simulink model "TuneWall"  (R2025b)
settings: Solver=VariableStepAuto  StartTime=0.0  StopTime=3600*4  RelTol=1e-3
model workspace (MAT data in the model file):
  h_in = 1.419
  h_out = 3.859
  k_Block = 0.01
  k_concrete = 0.11
libraries: fl_lib x66, nesl_utility x19, SimscapeFluids_lib x8
(part 2 of 2)

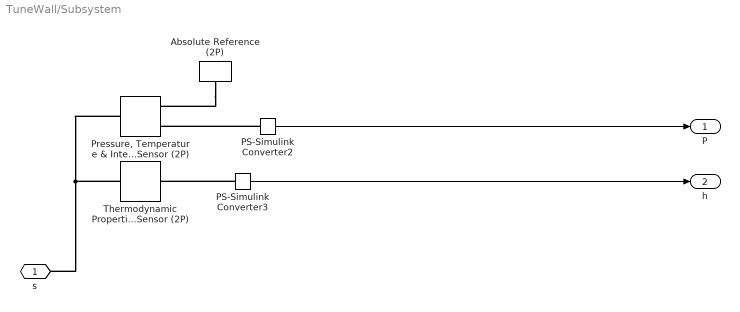
== system TuneWall/Subsystem ==
  Absolute Reference (2P) : fl_lib/Two-Phase Fluid/Elements/Absolute Reference (2P)
  PS-Simulink Converter2 : nesl_utility/PS-Simulink Converter  PhysicalDomain=network_engine_domain  SubClassName=ps_output  LeftPortType=input  RightPortType=output  PseudoPeriodic=off  Frequencies=[]  VectorFormat=inherit  Unit=inherit  AffineConversion=off
  PS-Simulink Converter3 : nesl_utility/PS-Simulink Converter  PhysicalDomain=network_engine_domain  SubClassName=ps_output  LeftPortType=input  RightPortType=output  PseudoPeriodic=off  Frequencies=[]  VectorFormat=inherit  Unit=inherit  AffineConversion=off
  "Pressure, Temperature & Internal Energy Sensor (2P)" : fl_lib/Two-Phase Fluid/Sensors/Pressure, Temperature & Internal Energy Sensor (2P)  reference=foundation.enum.MeasurementReference.difference  pressure=true  pressure_spec=foundation.enum.PressureMeasementSpec.Absolute  temperature=false  internal_energy=false
      settings: InternalSimscapePortConfiguration="{\"Bottom\":[],\"Left\":[{\"id\":\"A\",\"label\":\"A\",\"type\":\"foundation.two_phase_fluid.two_phase_fluid\"}],\"Right\":[{\"id\":\"B\",\"label\":\"B\",\"type\":\"foundation.two_phase_fluid.two_phase_fluid\"},{\"id\":\"P\",\"label\":\"P\",\"type\":\"output\"}],\"Top\":[]}"
  Thermodynamic Properties Sensor (2P) : fl_lib/Two-Phase Fluid/Sensors/Thermodynamic Properties Sensor (2P)  temperature=false  enthalpy=true  density=false  specific_volume=false  entropy=false
      settings: InternalSimscapePortConfiguration="{\"Bottom\":[],\"Left\":[{\"id\":\"A\",\"label\":\"A\",\"type\":\"foundation.two_phase_fluid.two_phase_fluid\"}],\"Right\":[{\"id\":\"H\",\"label\":\"h\",\"type\":\"output\"}],\"Top\":[]}"
  s : PMIOPort  Side=Left
  P : Outport
  h : Outport  Port=2
  wires:
  PS-Simulink Converter3/1 -> h/1
  PS-Simulink Converter2/1 -> P/1
  connections:
  Absolute Reference (2P)/LConn1 -- "Pressure, Temperature & Internal Energy Sensor (2P)"/RConn1
  PS-Simulink Converter2/LConn1 -- "Pressure, Temperature & Internal Energy Sensor (2P)"/RConn2
  PS-Simulink Converter3/LConn1 -- Thermodynamic Properties Sensor (2P)/RConn1
  "Pressure, Temperature & Internal Energy Sensor (2P)"/LConn1 -- s/RConn1 -- Thermodynamic Properties Sensor (2P)/LConn1

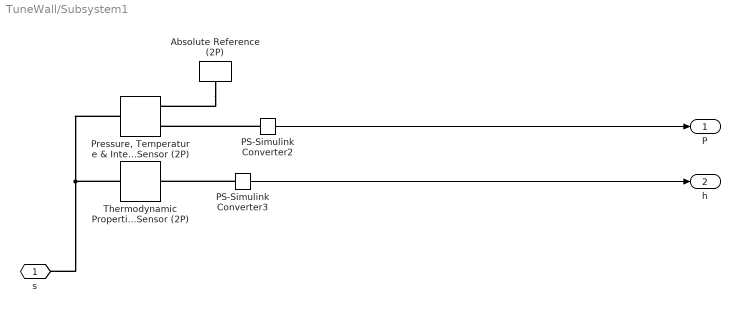
== system TuneWall/Subsystem1 ==
  Absolute Reference (2P) : fl_lib/Two-Phase Fluid/Elements/Absolute Reference (2P)
  PS-Simulink Converter2 : nesl_utility/PS-Simulink Converter  PhysicalDomain=network_engine_domain  SubClassName=ps_output  LeftPortType=input  RightPortType=output  PseudoPeriodic=off  Frequencies=[]  VectorFormat=inherit  Unit=inherit  AffineConversion=off
  PS-Simulink Converter3 : nesl_utility/PS-Simulink Converter  PhysicalDomain=network_engine_domain  SubClassName=ps_output  LeftPortType=input  RightPortType=output  PseudoPeriodic=off  Frequencies=[]  VectorFormat=inherit  Unit=inherit  AffineConversion=off
  "Pressure, Temperature & Internal Energy Sensor (2P)" : fl_lib/Two-Phase Fluid/Sensors/Pressure, Temperature & Internal Energy Sensor (2P)  reference=foundation.enum.MeasurementReference.difference  pressure=true  pressure_spec=foundation.enum.PressureMeasementSpec.Absolute  temperature=false  internal_energy=false
      settings: InternalSimscapePortConfiguration="{\"Bottom\":[],\"Left\":[{\"id\":\"A\",\"label\":\"A\",\"type\":\"foundation.two_phase_fluid.two_phase_fluid\"}],\"Right\":[{\"id\":\"B\",\"label\":\"B\",\"type\":\"foundation.two_phase_fluid.two_phase_fluid\"},{\"id\":\"P\",\"label\":\"P\",\"type\":\"output\"}],\"Top\":[]}"
  Thermodynamic Properties Sensor (2P) : fl_lib/Two-Phase Fluid/Sensors/Thermodynamic Properties Sensor (2P)  temperature=false  enthalpy=true  density=false  specific_volume=false  entropy=false
      settings: InternalSimscapePortConfiguration="{\"Bottom\":[],\"Left\":[{\"id\":\"A\",\"label\":\"A\",\"type\":\"foundation.two_phase_fluid.two_phase_fluid\"}],\"Right\":[{\"id\":\"H\",\"label\":\"h\",\"type\":\"output\"}],\"Top\":[]}"
  s : PMIOPort  Side=Left
  P : Outport
  h : Outport  Port=2
  wires:
  PS-Simulink Converter3/1 -> h/1
  PS-Simulink Converter2/1 -> P/1
  connections:
  Absolute Reference (2P)/LConn1 -- "Pressure, Temperature & Internal Energy Sensor (2P)"/RConn1
  PS-Simulink Converter2/LConn1 -- "Pressure, Temperature & Internal Energy Sensor (2P)"/RConn2
  PS-Simulink Converter3/LConn1 -- Thermodynamic Properties Sensor (2P)/RConn1
  "Pressure, Temperature & Internal Energy Sensor (2P)"/LConn1 -- Thermodynamic Properties Sensor (2P)/LConn1 -- s/RConn1

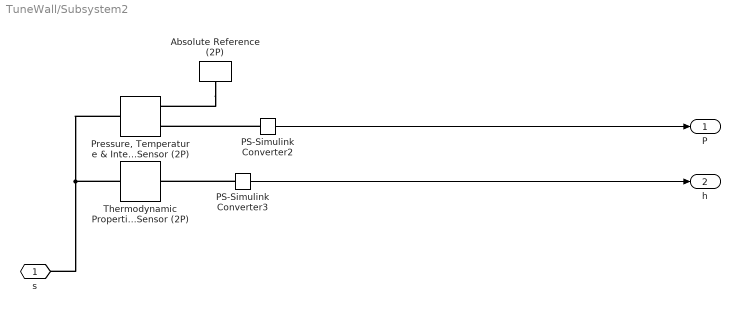
== system TuneWall/Subsystem2 ==
  Absolute Reference (2P) : fl_lib/Two-Phase Fluid/Elements/Absolute Reference (2P)
  PS-Simulink Converter2 : nesl_utility/PS-Simulink Converter  PhysicalDomain=network_engine_domain  SubClassName=ps_output  LeftPortType=input  RightPortType=output  PseudoPeriodic=off  Frequencies=[]  VectorFormat=inherit  Unit=inherit  AffineConversion=off
  PS-Simulink Converter3 : nesl_utility/PS-Simulink Converter  PhysicalDomain=network_engine_domain  SubClassName=ps_output  LeftPortType=input  RightPortType=output  PseudoPeriodic=off  Frequencies=[]  VectorFormat=inherit  Unit=inherit  AffineConversion=off
  "Pressure, Temperature & Internal Energy Sensor (2P)" : fl_lib/Two-Phase Fluid/Sensors/Pressure, Temperature & Internal Energy Sensor (2P)  reference=foundation.enum.MeasurementReference.difference  pressure=true  pressure_spec=foundation.enum.PressureMeasementSpec.Absolute  temperature=false  internal_energy=false
      settings: InternalSimscapePortConfiguration="{\"Bottom\":[],\"Left\":[{\"id\":\"A\",\"label\":\"A\",\"type\":\"foundation.two_phase_fluid.two_phase_fluid\"}],\"Right\":[{\"id\":\"B\",\"label\":\"B\",\"type\":\"foundation.two_phase_fluid.two_phase_fluid\"},{\"id\":\"P\",\"label\":\"P\",\"type\":\"output\"}],\"Top\":[]}"
  Thermodynamic Properties Sensor (2P) : fl_lib/Two-Phase Fluid/Sensors/Thermodynamic Properties Sensor (2P)  temperature=false  enthalpy=true  density=false  specific_volume=false  entropy=false
      settings: InternalSimscapePortConfiguration="{\"Bottom\":[],\"Left\":[{\"id\":\"A\",\"label\":\"A\",\"type\":\"foundation.two_phase_fluid.two_phase_fluid\"}],\"Right\":[{\"id\":\"H\",\"label\":\"h\",\"type\":\"output\"}],\"Top\":[]}"
  s : PMIOPort  Side=Left
  P : Outport
  h : Outport  Port=2
  wires:
  PS-Simulink Converter3/1 -> h/1
  PS-Simulink Converter2/1 -> P/1
  connections:
  Absolute Reference (2P)/LConn1 -- "Pressure, Temperature & Internal Energy Sensor (2P)"/RConn1
  PS-Simulink Converter2/LConn1 -- "Pressure, Temperature & Internal Energy Sensor (2P)"/RConn2
  PS-Simulink Converter3/LConn1 -- Thermodynamic Properties Sensor (2P)/RConn1
  "Pressure, Temperature & Internal Energy Sensor (2P)"/LConn1 -- Thermodynamic Properties Sensor (2P)/LConn1 -- s/RConn1

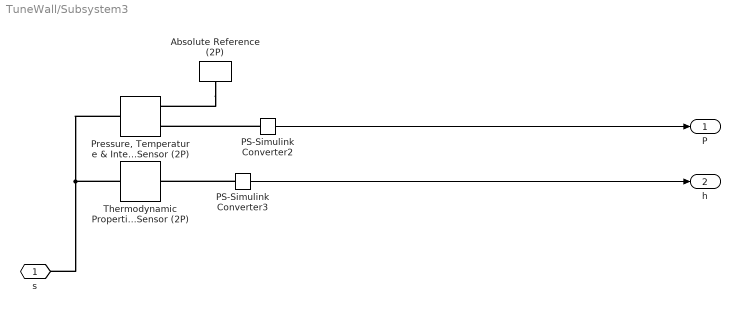
== system TuneWall/Subsystem3 ==
  Absolute Reference (2P) : fl_lib/Two-Phase Fluid/Elements/Absolute Reference (2P)
  PS-Simulink Converter2 : nesl_utility/PS-Simulink Converter  PhysicalDomain=network_engine_domain  SubClassName=ps_output  LeftPortType=input  RightPortType=output  PseudoPeriodic=off  Frequencies=[]  VectorFormat=inherit  Unit=inherit  AffineConversion=off
  PS-Simulink Converter3 : nesl_utility/PS-Simulink Converter  PhysicalDomain=network_engine_domain  SubClassName=ps_output  LeftPortType=input  RightPortType=output  PseudoPeriodic=off  Frequencies=[]  VectorFormat=inherit  Unit=inherit  AffineConversion=off
  "Pressure, Temperature & Internal Energy Sensor (2P)" : fl_lib/Two-Phase Fluid/Sensors/Pressure, Temperature & Internal Energy Sensor (2P)  reference=foundation.enum.MeasurementReference.difference  pressure=true  pressure_spec=foundation.enum.PressureMeasementSpec.Absolute  temperature=false  internal_energy=false
      settings: InternalSimscapePortConfiguration="{\"Bottom\":[],\"Left\":[{\"id\":\"A\",\"label\":\"A\",\"type\":\"foundation.two_phase_fluid.two_phase_fluid\"}],\"Right\":[{\"id\":\"B\",\"label\":\"B\",\"type\":\"foundation.two_phase_fluid.two_phase_fluid\"},{\"id\":\"P\",\"label\":\"P\",\"type\":\"output\"}],\"Top\":[]}"
  Thermodynamic Properties Sensor (2P) : fl_lib/Two-Phase Fluid/Sensors/Thermodynamic Properties Sensor (2P)  temperature=false  enthalpy=true  density=false  specific_volume=false  entropy=false
      settings: InternalSimscapePortConfiguration="{\"Bottom\":[],\"Left\":[{\"id\":\"A\",\"label\":\"A\",\"type\":\"foundation.two_phase_fluid.two_phase_fluid\"}],\"Right\":[{\"id\":\"H\",\"label\":\"h\",\"type\":\"output\"}],\"Top\":[]}"
  s : PMIOPort  Side=Left
  P : Outport
  h : Outport  Port=2
  wires:
  PS-Simulink Converter3/1 -> h/1
  PS-Simulink Converter2/1 -> P/1
  connections:
  Absolute Reference (2P)/LConn1 -- "Pressure, Temperature & Internal Energy Sensor (2P)"/RConn1
  PS-Simulink Converter2/LConn1 -- "Pressure, Temperature & Internal Energy Sensor (2P)"/RConn2
  PS-Simulink Converter3/LConn1 -- Thermodynamic Properties Sensor (2P)/RConn1
  "Pressure, Temperature & Internal Energy Sensor (2P)"/LConn1 -- Thermodynamic Properties Sensor (2P)/LConn1 -- s/RConn1

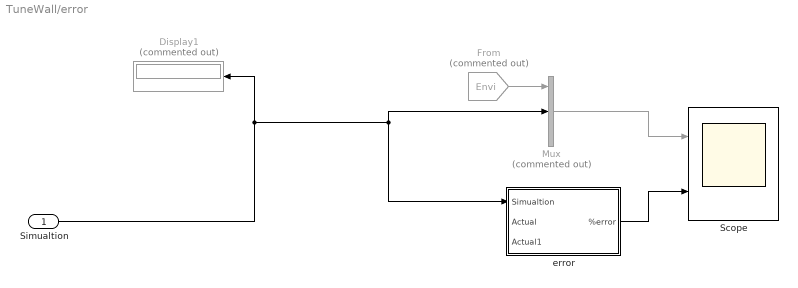
== system TuneWall/error ==
  Simualtion : Inport
  Display1 : Display  Commented=on
  From : From  Commented=on  GotoTag=Envi  TagVisibility=global
  Mux : Mux  Commented=on  Inputs=3
  Scope : Scope  NumInputPorts=2
      settings: Title=Error Sim vs Measurement  ActiveDisplayYMinimum=-100  ActiveDisplayYMaximum=100  YLabel=Error x100%
  error : Subsystem
  wires:
  Simualtion/1 -> Mux/2, error/1(Simualtion), Display1/1
  From/1 -> Mux/1
  Mux/1 -> Scope/1
  error/1(%error) -> Scope/2

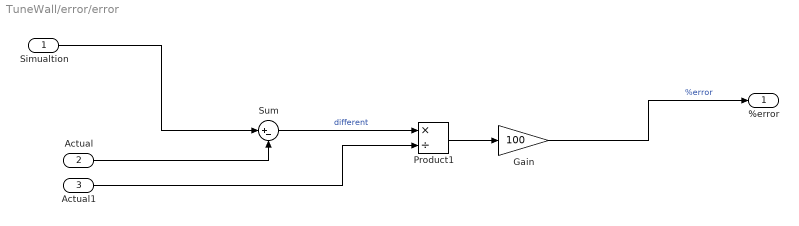
== system TuneWall/error/error ==
  Simualtion : Inport
  Actual : Inport  Port=2
  Actual1 : Inport  Port=3
  Gain : Gain  Gain=100
  Product1 : Product  Inputs=*/
  Sum : Sum  Inputs=|+-
  %error : Outport
  wires:
  Sum/1 -> Product1/1  "different"
  Product1/1 -> Gain/1
  Actual/1 -> Sum/2
  Gain/1 -> %error/1  "%error"
  Simualtion/1 -> Sum/1
  Actual1/1 -> Product1/2
